simulink model "s06_sig_template_25"  (R2025b)
settings: Solver=ode4  StopTime=inf  FixedStep=P_sim_dt  EnableMultiTasking=on
InitFcn:
  | s06_data;
values from neighbouring files (symbols this model uses):
  P_c_locate_problist = ones(P_car_cnt, 1, 'single')    [s06_data.m]
  P_display_dt = 50e-3    (= 0.05)    [s06_data.m]
  P_dt = 25e-3    (= 0.025)    [s06_data.m]
  P_p_aMax = 1    [baseline_lqr_script.m]    (also in d71_data.m)
  P_p_Bf = 0.7    [d01_data.m]
  P_p_Br = 0.7    [d01_data.m]
  P_p_Cf = 2    [d01_data.m]
  P_p_Cr = 2    [d01_data.m]
  P_p_delta_max = 21.58/180*pi    (= 0.37664205258)    [d01_data.m]    (also in d71_data.m = 0.383972435439)
  P_p_deltan_max = 1    [d01_data.m]    (also in d71_data.m = 0.93)
  P_p_deltan_min = -P_p_deltan_max    (= -1)    [d01_data.m]    (also in d71_data.m = -0.93)
  P_p_Df = 2    [d01_data.m]
  P_p_Dr = 2.5    [d01_data.m]
  P_p_Ef = -0.1    [d01_data.m]
  P_p_EG = 0    [d01_data.m]    (also in d71_data.m = 0.02)
  P_p_Er = -0.05    [d01_data.m]
  P_p_J = 192e-6    (= 0.000192)    [d01_data.m]    (also in d71_data.m = 3e-06)
  P_p_k = 2.51    [d01_data.m]    (also in d71_data.m = 3.4)
  P_p_kd0 = 0.04    [d71_data.m]
  P_p_kd1 = 0.15    [d71_data.m]
  P_p_l = abs(P_p_frontaxle_1 + P_p_rearaxle_1)    [d01_data.m]    (also in d71_data.m = 0.0325)
  P_p_lf = P_p_frontaxle_1    (= 0.05)    [d01_data.m]    (also in d71_data.m = 0.01625)
  P_p_lr = P_p_rearaxle_1    (= 0.049)    [d01_data.m]    (also in d71_data.m = 0.01625)
  P_p_m = 132e-3    (= 0.132)    [d01_data.m]    (also in d71_data.m = 0.013)
  P_p_T = 316e-3    (= 0.316)    [d01_data.m]    (also in d71_data.m = 0.12)
  P_p_Tt = P_p_uTt + P_p_output_Tt    (= 0.11)    [d01_data.m]    (also in d71_data.m = 0.1)
  P_p_un_max = 1    [d01_data.m]    (also in d71_data.m = 0.2)
  P_p_un_min = -P_p_un_max    (= -1)    [d01_data.m]    (also in d71_data.m = -0.2)
  P_p_vRef = 0.2    [baseline_lqr_script.m]    (also in d71_data.m = 0.15)
  P_p_xvec0 = [ P_p_v0; P_p_s10; P_p_s20; P_p_psi0; 0; 0; 0 ]    [d01_data.m]    (also in d71_data.m)
  P_p_xvec1 = [ P_p_v0; P_p_s11; P_p_s21; P_p_psi1; 0; 0; 0 ]    [d01_data.m]    (also in d71_data.m)
  P_vfilter = single([ 0.0 0.0 ... (first row only)    [s06_data.m]
undefined symbols (not defined in the file or in its folder): CarInputsCmdForward, DiscIntNeverNeededParam, ManeuverTypePark, ManeuverTypePathFollow, mbc_car_display, P_cpseq, P_p, P_track
libraries: vrlib x2
(part 1 of 2)
settings Model: Creator=ftraenkle  LastModifiedBy=jossie
settings SolverCC: AlgebraicLoopSolver=TrustRegion
settings DataIOCC: LimitDataPoints=on  InspectSignalLogs=on  ReturnWorkspaceOutputs=off
settings OptimizationCC: DefaultParameterBehavior=Inlined  EnhancedBackFolding=on  PassReuseOutputArgsAs=Individual arguments  ExpressionDepthLimit=2147483647.0  ZeroExternalMemoryAtStartup=off  ZeroInternalMemoryAtStartup=off  OptimizeBlockOrder=speed  DifferentSizesBufferReuse=on  OptimizationCustomize=off  EfficientTunableParamExpr=on
settings DebuggingCC: SolverPrmCheckMsg=warning  ParameterTunabilityLossMsg=error  UnconnectedInputMsg=warning  UnconnectedOutputMsg=warning  UnconnectedLineMsg=warning  BusObjectLabelMismatch=error  AllowSymbolicDim=off  StateNameClashWarn=warning  SFUnexpectedBacktrackingDiag=warning  SFNoUnconditionalDefaultTransitionDiag=warning  SFExecutionAtInitializationDiag=none  ArithmeticOperatorsInVariantConditions=warning
settings HardwareCC: ProdBitPerLong=64.0  ProdHWDeviceType=Intel->x86-64 (Linux 64)
settings ModelReferenceCC: EnableRefExpFcnMdlSchedulingChecks=on
settings SFSimCC: SimUseLocalCustomCode=off  CustomCodeUndefinedFunction=UseInterfaceOnly
settings RTWCC: SystemTargetFile=ert.tlc  GenCodeOnly=on  PackageGeneratedCodeAndArtifacts=on  PackageName=d1.zip  TemplateMakefile=ert_default_tmf  GenerateReport=on  RTWUseLocalCustomCode=off  IncludeHyperlinkInReport=on  GenerateTraceInfo=on  GenerateTraceReportEml=on  GPUComputeCapability=3.5  DLArmComputeVersion=19.05  Description=Embedded Coder
settings CodeAppCC: ForceParamTrailComments=on  IgnoreCustomStorageClasses=off  OperatorAnnotations=on  SimulinkDataObjDesc=on  SFDataObjDesc=on  InsertBlockDesc=on
settings ERTTargetCC: RootIOFormat=Structure reference  DynamicArrayContainerType=coder::array  SupportVariableSizeSignals=on
settings ConfigComp: CovMetricSettings=dw  CovSaveCumulativeToWorkspaceVar=on  CovSaveSingleToWorkspaceVar=on  CovExternalEMLEnable=off

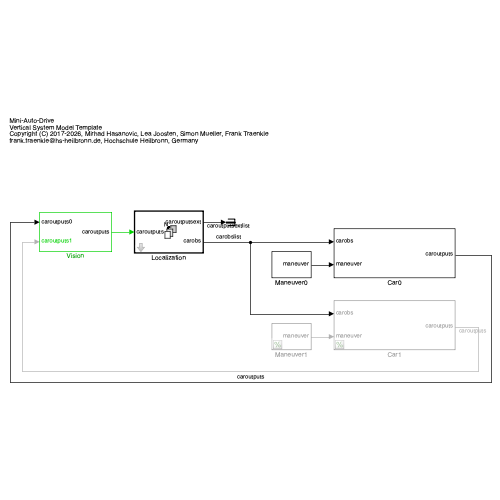
[thumbnail: Simulink's stored preview of the top-level diagram]
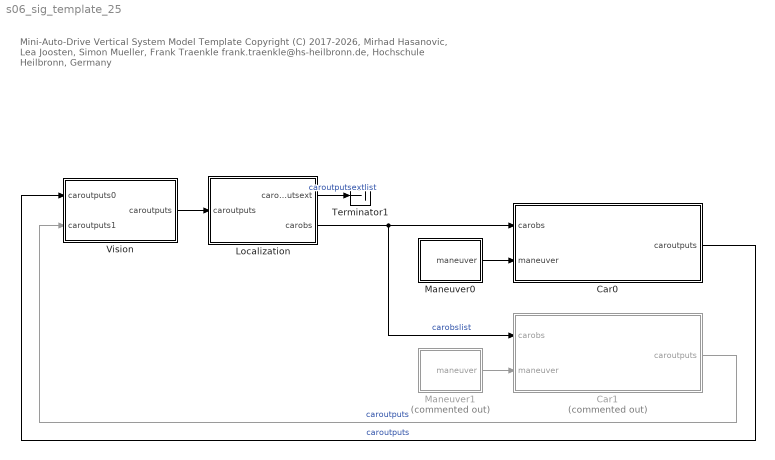
== system s06_sig_template_25 ==
  note: Mini-Auto-Drive
      | Vertical System Model Template
      | Copyright (C) 2017-2026, Mirhad Hasanovic, Lea Joosten, Simon Mueller, Frank Traenkle
      | frank.traenkle@hs-heilbronn.de, Hochschule Heilbronn, Germany
  Car0 : Subsystem
  Car1 : Subsystem  Commented=on
  Localization : Subsystem  TreatAsAtomicUnit=on  mask{P_mask_problist=P_c_locate_problist}
      mask prompts: P_mask_problist "Locate Probability"
  Maneuver0 : Subsystem
  Maneuver1 : Subsystem  Commented=on
  Terminator1 : Terminator
  Vision : Subsystem
  wires:
  Car0/1(caroutputs) -> Vision/1(caroutputs0)  "caroutputs"
  Localization/2(carobs) -> Car1/1(carobs), Car0/1(carobs)  "carobslist"
  Vision/1(caroutputs) -> Localization/1(caroutputs)
  Car1/1(caroutputs) -> Vision/2(caroutputs1)  "caroutputs"
  Maneuver0/1(maneuver) -> Car0/2(maneuver)
  Maneuver1/1(maneuver) -> Car1/2(maneuver)
  Localization/1(caroutputsext) -> Terminator1/1  "caroutputsextlist"

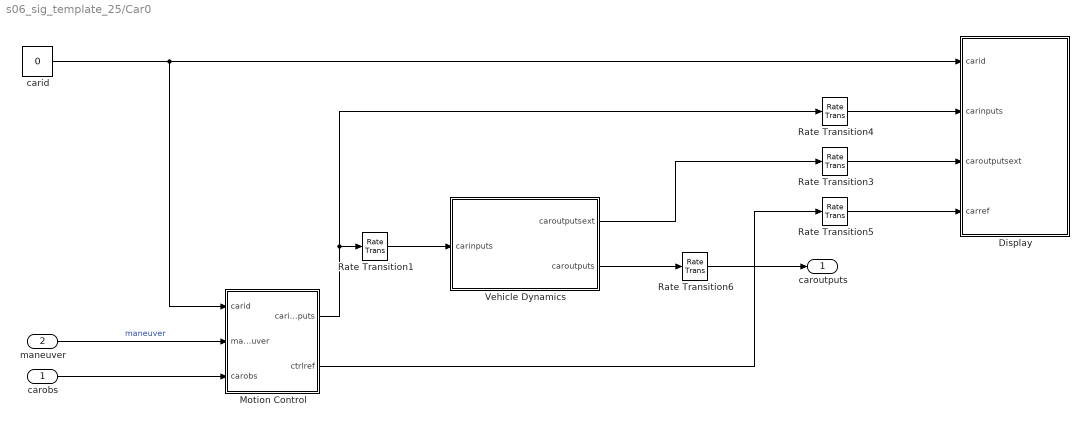
== system s06_sig_template_25/Car0 ==
  carobs : Inport  OutDataTypeStr=Bus: CAROBS
  maneuver : Inport  Port=2
  Display : Subsystem  TreatAsAtomicUnit=on  SystemSampleTime=P_display_dt
  Motion Control : Subsystem  TreatAsAtomicUnit=on
  Rate Transition1 : RateTransition  Integrity=off
  Rate Transition{3..6} (4 alike) : RateTransition
  Vehicle Dynamics : Subsystem  mask{P_mask_vec0=P_p_xvec0, P_mask_p=P_p(1)}
      mask prompts: P_mask_vec0 "Initial value"; P_mask_p "Parameters"
  carid : Constant  Value=0
  caroutputs : Outport  OutDataTypeStr=Bus: CAROUTPUTS
  wires:
  Vehicle Dynamics/1(caroutputsext) -> Rate Transition3/1
  Rate Transition5/1 -> Display/4(carref)
  Rate Transition3/1 -> Display/3(caroutputsext)
  Rate Transition4/1 -> Display/2(carinputs)
  Rate Transition1/1 -> Vehicle Dynamics/1(carinputs)
  Vehicle Dynamics/2(caroutputs) -> Rate Transition6/1
  Rate Transition6/1 -> caroutputs/1
  carid/1 -> Motion Control/1(carid), Display/1(carid)
  Motion Control/1(carinputs) -> Rate Transition4/1, Rate Transition1/1
  Motion Control/2(ctrlref) -> Rate Transition5/1
  carobs/1 -> Motion Control/3(carobs)
  maneuver/1 -> Motion Control/2(maneuver)  "maneuver"

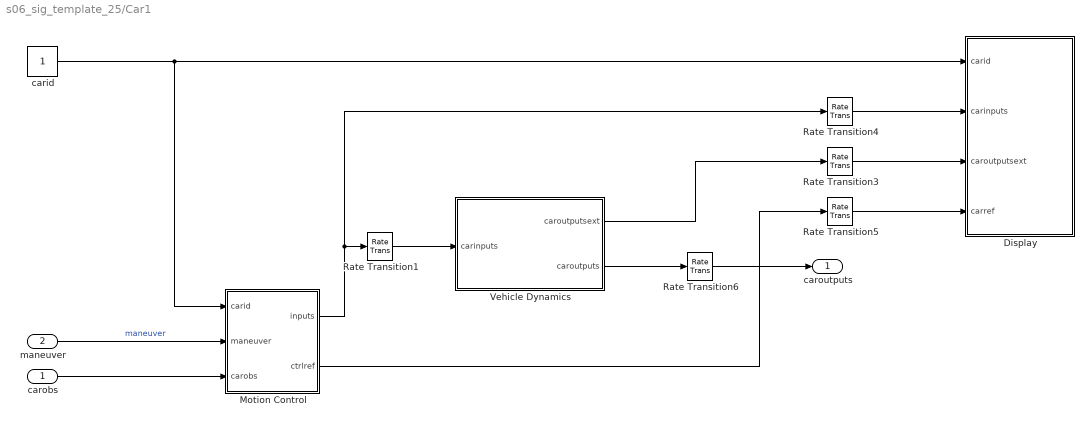
== system s06_sig_template_25/Car1 ==
  carobs : Inport  OutDataTypeStr=Bus: CAROBS
  maneuver : Inport  Port=2
  Display : Subsystem  TreatAsAtomicUnit=on  SystemSampleTime=P_display_dt
  Motion Control : Subsystem  TreatAsAtomicUnit=on  SystemSampleTime=P_dt
  Rate Transition{1,3..6} (5 alike) : RateTransition
  Vehicle Dynamics : Subsystem  mask{P_mask_vec0=P_p_xvec1, P_mask_p=P_p(1)}
      mask prompts: P_mask_vec0 "Initial value"; P_mask_p "Parameters"
  carid : Constant
  caroutputs : Outport  OutDataTypeStr=Bus: CAROUTPUTS
  wires:
  Vehicle Dynamics/1(caroutputsext) -> Rate Transition3/1
  Rate Transition5/1 -> Display/4(carref)
  Rate Transition3/1 -> Display/3(caroutputsext)
  Rate Transition4/1 -> Display/2(carinputs)
  Rate Transition1/1 -> Vehicle Dynamics/1(carinputs)
  Vehicle Dynamics/2(caroutputs) -> Rate Transition6/1
  Rate Transition6/1 -> caroutputs/1
  carid/1 -> Motion Control/1(carid), Display/1(carid)
  Motion Control/1(inputs) -> Rate Transition4/1, Rate Transition1/1
  Motion Control/2(ctrlref) -> Rate Transition5/1
  carobs/1 -> Motion Control/3(carobs)
  maneuver/1 -> Motion Control/2(maneuver)  "maneuver"

== system s06_sig_template_25/Localization ==
  caroutputs : Inport  Partition=on  PartitionDimension=1  PartitionWidth=1  PartitionOffset=0
  Constant : Constant  Value=true
  For Each : ForEach  DisableCoverage=on  IterateSubsysMaskParameter=on
  Locate : Subsystem
  caroutputsext : Outport  ConcatenationDimension=1
  carobs : Outport  Port=2  ConcatenationDimension=1
  wires:
  Locate/1(caroutputsext) -> caroutputsext/1
  Constant/1 -> Locate/Enable
  caroutputs/1 -> Locate/1(caroutputs)
  Locate/2(carobs) -> carobs/1

== system s06_sig_template_25/Maneuver0 ==
  Constant : Constant  Value=ManeuverTypePark
  Constant1 : Constant  Value=single(0.4)
  Constant2 : Constant  Value=single(2.0)
  Create Maneuver : MATLAB Function  TreatAsAtomicUnit=on
  maneuver : Outport
  wires:
  Constant/1 -> Create Maneuver/1(type)
  Constant1/1 -> Create Maneuver/2(vmax)
  Constant2/1 -> Create Maneuver/3(xref)
  Create Maneuver/1(maneuver) -> maneuver/1  "maneuver"

== system s06_sig_template_25/Maneuver1 ==
  Constant : Constant  Value=ManeuverTypePathFollow
  Constant1 : Constant  Value=single(0.5)
  Constant2 : Constant  Value=single(1.0)
  Create Maneuver : MATLAB Function  TreatAsAtomicUnit=on
  maneuver : Outport
  wires:
  Create Maneuver/1(maneuver) -> maneuver/1  "maneuver"
  Constant2/1 -> Create Maneuver/3(xref)
  Constant1/1 -> Create Maneuver/2(vmax)
  Constant/1 -> Create Maneuver/1(type)

== system s06_sig_template_25/Vision ==
  caroutputs0 : Inport  OutDataTypeStr=Bus:CAROUTPUTS
  caroutputs1 : Inport  Port=2  OutDataTypeStr=Bus:CAROUTPUTS
  Vector Concatenate : Concatenate  NumInputs=P_car_cnt
  caroutputs : Outport  OutDataTypeStr=Bus:CAROUTPUTS
  wires:
  Vector Concatenate/1 -> caroutputs/1  "caroutputs"
  caroutputs0/1 -> Vector Concatenate/1
  caroutputs1/1 -> Vector Concatenate/2

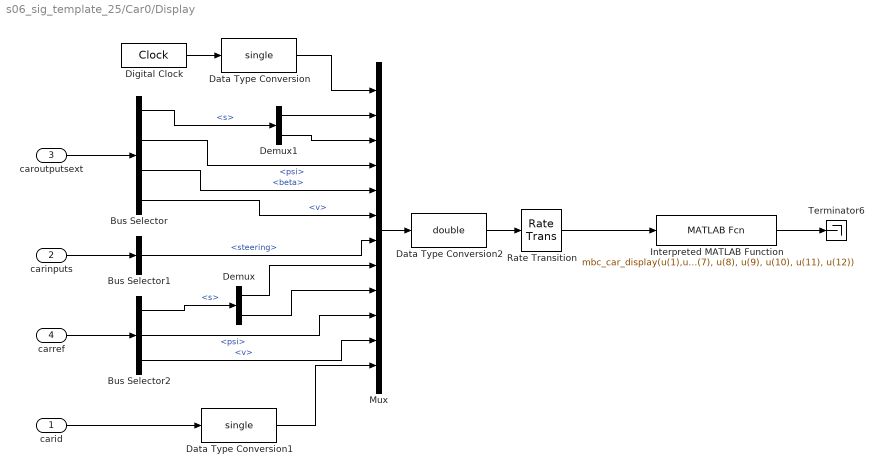
== system s06_sig_template_25/Car0/Display ==
  carid : Inport
  carinputs : Inport  Port=2
  caroutputsext : Inport  Port=3
  carref : Inport  Port=4
  Bus Selector : BusSelector  OutputSignals=s,psi,beta,v
  Bus Selector1 : BusSelector  OutputSignals=steering
  Bus Selector2 : BusSelector  OutputSignals=s,psi,v
  Data Type Conversion : DataTypeConversion  OutDataTypeStr=single  SaturateOnIntegerOverflow=off  RndMeth=Floor
  Data Type Conversion1 : DataTypeConversion  OutDataTypeStr=single  SaturateOnIntegerOverflow=off  RndMeth=Floor
  Data Type Conversion2 : DataTypeConversion  OutDataTypeStr=double  SaturateOnIntegerOverflow=off  RndMeth=Floor
  Demux : Demux  Outputs=2
  Demux1 : Demux  Outputs=2
  Digital Clock : DigitalClock  SampleTime=-1
  Interpreted MATLAB Function : MATLABFcn  MATLABFcn=mbc_car_display(u(1),u(2),u(3),u(4),u(5), u(6), u(7), u(8), u(9), u(10), u(11), u(12))
  Mux : Mux  Inputs=12
  Rate Transition : RateTransition  OutPortSampleTime=P_display_dt
  Terminator6 : Terminator
  wires:
  caroutputsext/1 -> Bus Selector/1
  Interpreted MATLAB Function/1 -> Terminator6/1
  Mux/1 -> Data Type Conversion2/1
  Rate Transition/1 -> Interpreted MATLAB Function/1
  Digital Clock/1 -> Data Type Conversion/1
  Bus Selector/2 -> Mux/4  "<psi>"
  carinputs/1 -> Bus Selector1/1
  Bus Selector1/1 -> Mux/7  "<steering>"
  Bus Selector/3 -> Mux/5  "<beta>"
  Bus Selector/4 -> Mux/6  "<v>"
  carref/1 -> Bus Selector2/1
  Bus Selector2/3 -> Mux/11  "<v>"
  Bus Selector2/2 -> Mux/10  "<psi>"
  Bus Selector2/1 -> Demux/1  "<s>"
  carid/1 -> Data Type Conversion1/1
  Data Type Conversion/1 -> Mux/1
  Data Type Conversion1/1 -> Mux/12
  Data Type Conversion2/1 -> Rate Transition/1
  Demux/1 -> Mux/8
  Demux/2 -> Mux/9
  Bus Selector/1 -> Demux1/1  "<s>"
  Demux1/1 -> Mux/2
  Demux1/2 -> Mux/3

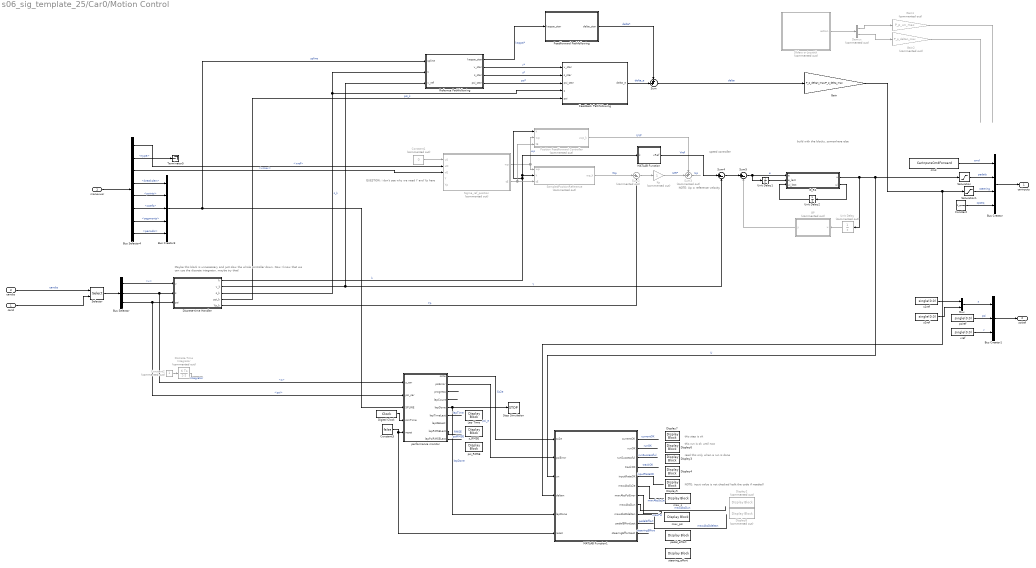
== system s06_sig_template_25/Car0/Motion Control ==
  note: Maybe this block is unnecessary and just slow the whole controller down. Now I know that we can use the discrete integrator, maybe try that!
  note: build with the blocks, somewhere else
  note: speed controller
  note: NOTE: Up = reference velocity
  note: QUESTION: i don't see why we need Y and Yp here
  note: read this only when a run is done
  note: NOTE: input value is not checked (edit the code if needed)
  note: this run is ok until now
  note: this step is ok
  carid : Inport
  maneuver : Inport  Port=2
  carobs : Inport  Port=3
  Bus Creator : BusCreator  Inputs=4  OutDataTypeStr=Bus: CARINPUTS  NonVirtualBus=on
  Bus Creator1 : BusCreator  Inputs=3  OutDataTypeStr=Bus: CTRLREFERENCE  NonVirtualBus=on
  Bus Creator3 : BusCreator  Inputs=5  OutDataTypeStr=Bus: SPLINE
  Bus Selector : BusSelector  OutputSignals=v,s,psi
  Bus Selector4 : BusSelector  OutputSignals=xref,type,vmax,breakslen,points,coefs,segments,periodic
  Constant : Constant  Value=P_cpseq  OutDataTypeStr=Bus: CHECKPOINTSEQUENCEMSG
  Constant1 : Constant  Commented=on  Value=0
  Constant2 : Constant  Commented=on
  Constant3 : Constant  Value=false
  Demux : Demux  Commented=on  Outputs=2
  Digital Clock : DigitalClock  SampleTime=P_dt
  Discrete-Time Integrator : DiscreteIntegrator  Commented=on  SampleTime=0.025  ICPrevOutput=DiscIntNeverNeededParam  ICPrevScaledInput=DiscIntNeverNeededParam
  Discrete-time Handler : MATLAB Function  TreatAsAtomicUnit=on
  Display2 : DisplayBlock  Commented=on  LabelPosition=Hide  Transparency=1  GridColor=[0.502, 0.502, 0.502]
  Display{3..7} (5 alike) : DisplayBlock  LabelPosition=Hide  Transparency=1  GridColor=[0.502, 0.502, 0.502]
  Display8 : DisplayBlock  Commented=on  LabelPosition=Hide  Transparency=1  GridColor=[0.502, 0.502, 0.502]
  Feedback Pathfollowing : MATLAB Function  TreatAsAtomicUnit=on
  Feedforward Pathfollowing : MATLAB Function  TreatAsAtomicUnit=on
  GP : MATLAB Function  Commented=on  TreatAsAtomicUnit=on
  G_R1 : MATLAB Function  TreatAsAtomicUnit=on
  Gain : Gain  Gain=P_p_deltan_max/P_p_delta_max
  Gain1 : Gain  Commented=on  Gain=P_p_un_max
  Gain2 : Gain  Commented=on  Gain=P_p_deltan_max
  Kp : Gain  Commented=on
  Lap Time : DisplayBlock  LabelPosition=Hide  Transparency=1  GridColor=[0.502, 0.502, 0.502]
  MATLAB Function : MATLAB Function  TreatAsAtomicUnit=on
  MATLAB Function1 : MATLAB Function  TreatAsAtomicUnit=on
  Mux : Mux  Inputs=2
  Position Feedforward Controller : MATLAB Function  Commented=on  TreatAsAtomicUnit=on
  Refernce Pathfollowing : MATLAB Function  TreatAsAtomicUnit=on
  SampledPositionReference : MATLAB Function  Commented=on  TreatAsAtomicUnit=on
  Saturation : Saturate  UpperLimit=P_p_un_max  LowerLimit=P_p_un_min
  Saturation1 : Saturate  UpperLimit=P_p_deltan_max  LowerLimit=P_p_deltan_min
  Selector : Selector  IndexMode=Zero-based  InputPortWidth=P_car_cnt  IndexOptions=Index vector (port)  Indices=0  OutputSizes=1
  Sigma_ref_position : MATLAB Function  Commented=on  TreatAsAtomicUnit=on
  Sliders or Joystick : Subsystem  Commented=on  Variant=on  VariantControlMode=label  LabelModeActiveChoice=true
  Stop Simulation : Stop
  Sum : Sum  Inputs=++|
  Sum2 : Sum  Commented=on  Inputs=|+-
  Sum3 : Sum  Commented=on  Inputs=++|
  Sum4 : Sum  Inputs=|+-
  Sum5 : Sum  Inputs=|+-
  Terminator5 : Terminator
  Unit Delay : UnitDelay  Commented=on  SampleTime=-1
  Unit Delay1 : UnitDelay  SampleTime=-1
  Unit Delay2 : UnitDelay  SampleTime=-1
  cmd : Constant  Value=CarInputsCmdForward
  max_psi : DisplayBlock  LabelPosition=Hide  Transparency=1  GridColor=[0.502, 0.502, 0.502]
  max_s : DisplayBlock  LabelPosition=Hide  Transparency=1  GridColor=[0.502, 0.502, 0.502]
  pedal_effort : DisplayBlock  LabelPosition=Hide  Transparency=1  GridColor=[0.502, 0.502, 0.502]
  performance monitor : MATLAB Function  TreatAsAtomicUnit=on
  psi_RMSE : DisplayBlock  LabelPosition=Hide  Transparency=1  GridColor=[0.502, 0.502, 0.502]
  psiref : Constant  Value=single(0.0)
  s1ref : Constant  Value=single(0.0)
  s2ref : Constant  Value=single(0.0)
  s_RMSE : DisplayBlock  LabelPosition=Hide  Transparency=1  GridColor=[0.502, 0.502, 0.502]
  steering_effort : DisplayBlock  LabelPosition=Hide  Transparency=1  GridColor=[0.502, 0.502, 0.502]
  vref : Constant  Value=single(0.0)
  carinputs : Outport  VectorParamsAs1DForOutWhenUnconnected=off
  ctrlref : Outport  Port=2  VectorParamsAs1DForOutWhenUnconnected=off
  wires:
  Bus Creator1/1 -> ctrlref/1
  vref/1 -> Bus Creator1/3  "v"
  Bus Selector/2 -> performance monitor/1(s_car), Discrete-time Handler/2(s)  "<s>"
  Mux/1 -> Bus Creator1/1  "s"
  Bus Selector4/7 -> Bus Creator3/4  "<segments>"
  Bus Selector4/5 -> Bus Creator3/2  "<points>"
  Bus Selector4/6 -> Bus Creator3/3  "<coefs>"
  Bus Selector4/8 -> Bus Creator3/5  "<periodic>"
  Bus Selector4/2 -> Terminator5/1  "<type>"
  Bus Selector4/4 -> Bus Creator3/1  "<breakslen>"
  maneuver/1 -> Bus Selector4/1
  carid/1 -> Selector/2
  carobs/1 -> Selector/1  "carobs"
  Selector/1 -> Bus Selector/1
  Bus Selector4/1 -> Sigma_ref_position/2(xD)  "<xref>"
  Bus Selector4/3 -> Sigma_ref_position/3(vE)  "<vmax>"
  Bus Selector/1 -> Discrete-time Handler/1(v)  "<v>"
  Bus Selector/3 -> performance monitor/2(psi_car), Discrete-time Handler/3(psi)  "<psi>"
  s1ref/1 -> Mux/1
  s2ref/1 -> Mux/2
  psiref/1 -> Bus Creator1/2  "psi"
  Demux/1 -> Gain1/1
  Constant/1 -> Bus Creator/4  "cpseq"
  Bus Creator/1 -> carinputs/1
  cmd/1 -> Bus Creator/1  "cmd"
  Gain1/1 -> ?
  Saturation1/1 -> Bus Creator/3  "steering"
  Sliders or Joystick/1(action) -> Demux/1
  Demux/2 -> Gain2/1
  Gain2/1 -> ?
  Saturation/1 -> Bus Creator/2  "pedals"
  Bus Creator3/1 -> performance monitor/3(SPLINE), Refernce Pathfollowing/1(spline)  "spline"
  Constant1/1 -> Sigma_ref_position/1(v0)
  SampledPositionReference/1(wp_k) -> Sum2/1  "Wp"
  Sigma_ref_position/1(wp) -> Position Feedforward Controller/2(wp), SampledPositionReference/1(wp)  "wp"
  Discrete-time Handler/1(k) -> MATLAB Function/1(k), SampledPositionReference/2(k), Position Feedforward Controller/1(k)  "k"
  Discrete-time Handler/5(Yp_k) -> Sum2/2  "Yp"
  Sum2/1 -> Kp/1
  Kp/1 -> Sum3/2  "URP"
  Sum3/1 -> ?  "Up"
  Position Feedforward Controller/1(uvp_k) -> Sum3/1  "UVP"
  Discrete-time Handler/2(v_k) -> Refernce Pathfollowing/3(v_ref), Sum4/2  "Y"
  Sum4/1 -> Sum5/1
  GP/1(y) -> Sum5/2
  Sum5/1 -> Unit Delay1/1, G_R1/1(e)  "e"
  Unit Delay1/1 -> G_R1/2(e_last)
  G_R1/2(ui) -> Unit Delay2/1
  Unit Delay2/1 -> G_R1/3(ui_last)
  Feedforward Pathfollowing/1(delta_star) -> Sum/1  "delta*"
  Feedback Pathfollowing/1(delta_e) -> Sum/2  "delta_e"
  Refernce Pathfollowing/1(kappa_star) -> Feedforward Pathfollowing/1(kappa_star)  "kappa*"
  Refernce Pathfollowing/2(v_star) -> Feedback Pathfollowing/1(v_star)  "v*"
  Refernce Pathfollowing/3(s_star) -> Feedback Pathfollowing/2(s_star)  "s*"
  Refernce Pathfollowing/4(psi_star) -> Feedback Pathfollowing/3(psi_star)  "psi*"
  Discrete-time Handler/3(s_k) -> Refernce Pathfollowing/2(s), Feedback Pathfollowing/4(s)  "s_k"
  Discrete-time Handler/4(psi_k) -> Feedback Pathfollowing/5(psi)  "psi_k"
  Sum/1 -> Gain/1  "delta"
  Unit Delay/1 -> GP/1(u)
  Constant2/1 -> Discrete-Time Integrator/1
  Discrete-Time Integrator/1 -> ?  "integrator"
  Sigma_ref_position/2(tE) -> SampledPositionReference/3(tE), Position Feedforward Controller/3(tE)
  Gain/1 -> MATLAB Function1/4(deltan), Saturation1/1
  MATLAB Function/1(vRef) -> Sum4/1  "Vref"
  MATLAB Function1/9(maxAbsDdeltan) -> ?  "maxAbsDdeltan"
  MATLAB Function1/8(maxAbsDun) -> ?  "maxAbsDun"
  Constant3/1 -> MATLAB Function1/6(reset), performance monitor/5(reset)
  performance monitor/5(lapDone) -> Stop Simulation/1, MATLAB Function1/5(lapDone)  "lapDone"
  G_R1/1(u) -> Saturation/1, MATLAB Function1/3(un), Unit Delay/1  "U"
  MATLAB Function1/3(runSuccessful) -> ?  "runSuccessful"
  performance monitor/1(sc2e) -> MATLAB Function1/1(sc2e)  "Sc2e"
  performance monitor/2(psiError) -> MATLAB Function1/2(psiError)  "psi_e"
  performance monitor/9(lapPsiRMSELast) -> ?  "psiRMSE"
  MATLAB Function1/2(runOK) -> ?  "runOK"
  MATLAB Function1/10(pedalEffortLast) -> ?  "pedalEffort"
  MATLAB Function1/11(steeringEffortLast) -> ?  "steeringEffort"
  MATLAB Function1/7(maxAbsPsiError) -> ?  "maxPsi"
  MATLAB Function1/1(currentOK) -> ?  "currentOK"
  Digital Clock/1 -> performance monitor/4(simTime)
  MATLAB Function1/5(inputRateOK) -> ?  "inputRateOK"
  performance monitor/4(lapCount) -> ?
  MATLAB Function1/4(trackOK) -> ?  "trackOK"
  MATLAB Function1/6(maxAbsSc2e) -> ?  "maxAbsSc2e"
  performance monitor/6(lapTimeLast) -> ?  "lapTime"
  performance monitor/3(progress) -> ?
  performance monitor/8(lapRMSELast) -> ?  "RMSE"

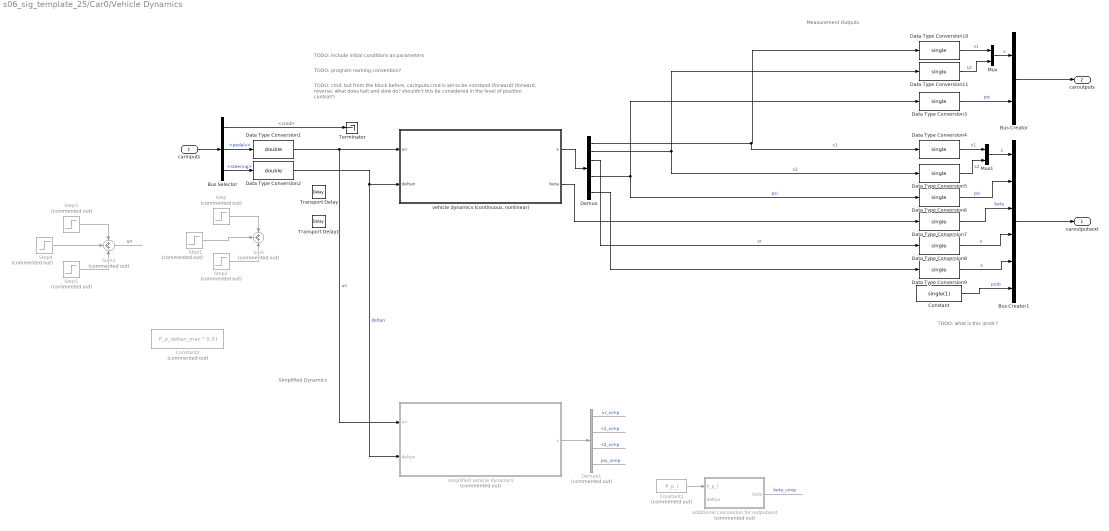
== system s06_sig_template_25/Car0/Vehicle Dynamics ==
  note: Simplified Dynamics
  note: TODO: cmd, but from the block before, carinputs.cmd is set to be constand (forward)
      | (forward, reverse, what does halt and slow do? shouldn't this be considered in the level of position control?)
  note: TODO: what is this 'prob'?
  note: TODO: program naming convention?
  note: TODO: include initial conditions as parameters
  note: Measurement Outputs
  carinputs : Inport
  Bus Creator : BusCreator  Inputs=2  OutDataTypeStr=Bus: CAROUTPUTS  NonVirtualBus=on
  Bus Creator1 : BusCreator  Inputs=6  OutDataTypeStr=Bus: CAROUTPUTSEXT  NonVirtualBus=on
  Bus Selector : BusSelector  OutputSignals=cmd,pedals,steering
  Constant : Constant  Value=single(1)
  Constant1 : Constant  Commented=on  Value=P_p_l
  Constant2 : Constant  Commented=on  Value=P_p_deltan_max * 0.01
  Data Type Conversion1 : DataTypeConversion  OutDataTypeStr=double  SaturateOnIntegerOverflow=off  RndMeth=Floor
  Data Type Conversion{3..11} (9 alike) : DataTypeConversion  OutDataTypeStr=single  SaturateOnIntegerOverflow=off  RndMeth=Floor
  Data Type Conversion2 : DataTypeConversion  OutDataTypeStr=double  SaturateOnIntegerOverflow=off  RndMeth=Floor
  Demux : Demux  Outputs=7
  Demux1 : Demux  Commented=on
  Mux : Mux  Inputs=2
  Mux1 : Mux  Inputs=2
  Step : Step  Commented=on  Time=0  After=P_p_un_max*0.5  SampleTime=0
  Step1 : Step  Commented=on  After=-P_p_un_max*0.5  SampleTime=0
  Step2 : Step  Commented=on  Time=2  After=P_p_un_max  SampleTime=0
  Step3 : Step  Commented=on  Time=0  After=P_p_un_max  SampleTime=0
  Step4 : Step  Commented=on  After=-2*P_p_un_max  SampleTime=0
  Step5 : Step  Commented=on  Time=2  After=P_p_un_max  SampleTime=0
  Sum : Sum  Commented=on  Inputs=+++
  Sum1 : Sum  Commented=on  Inputs=+++
  Terminator : Terminator
  Transport Delay : TransportDelay  DelayTime=P_p_Tt
  Transport Delay1 : TransportDelay  DelayTime=P_p_Tt
  additional calculation for outputsext : MATLAB Function  Commented=on  TreatAsAtomicUnit=on
  simplified vehicle dynamics : Subsystem  Commented=on
  "vehicle dynamics (continuous, nonlinear)" : Subsystem
  caroutputsext : Outport  OutDataTypeStr=Bus: CAROUTPUTSEXT  VectorParamsAs1DForOutWhenUnconnected=off
  caroutputs : Outport  Port=2  OutDataTypeStr=Bus: CAROUTPUTS  VectorParamsAs1DForOutWhenUnconnected=off
  wires:
  Bus Selector/2 -> Data Type Conversion1/1  "<pedals>"
  Bus Selector/3 -> Data Type Conversion2/1  "<steering>"
  Bus Creator/1 -> caroutputs/1
  Bus Creator1/1 -> caroutputsext/1
  Bus Selector/1 -> Terminator/1  "<cmd>"
  Mux1/1 -> Bus Creator1/1  "s"
  Data Type Conversion5/1 -> Mux1/2  "s2"
  Data Type Conversion4/1 -> Mux1/1  "s1"
  Mux/1 -> Bus Creator/1  "s"
  Data Type Conversion9/1 -> Bus Creator1/5  "x"
  Data Type Conversion8/1 -> Bus Creator1/4  "v"
  Data Type Conversion7/1 -> Bus Creator1/3  "beta"
  Data Type Conversion6/1 -> Bus Creator1/2  "psi"
  Data Type Conversion3/1 -> Bus Creator/2  "psi"
  Data Type Conversion11/1 -> Mux/2  "s2"
  Data Type Conversion10/1 -> Mux/1  "s1"
  Constant/1 -> Bus Creator1/6  "prob"
  "vehicle dynamics (continuous, nonlinear)"/1(x) -> Demux/1
  Demux/1 -> Data Type Conversion4/1, Data Type Conversion10/1  "s1"
  Demux/2 -> Data Type Conversion5/1, Data Type Conversion11/1  "s2"
  Demux/5 -> Data Type Conversion6/1, Data Type Conversion3/1  "psi"
  "vehicle dynamics (continuous, nonlinear)"/2(beta) -> Data Type Conversion7/1
  Demux/7 -> Data Type Conversion9/1
  Demux/3 -> Data Type Conversion8/1  "vr"
  simplified vehicle dynamics/1(x) -> Demux1/1
  Demux1/1 -> ?  "vr_simp"
  Constant1/1 -> additional calculation for outputsext/1(P_p_l)
  Demux1/2 -> ?  "s1_simp"
  Demux1/3 -> ?  "s2_simp"
  Demux1/4 -> ?  "psi_simp"
  additional calculation for outputsext/1(beta) -> ?  "beta_simp"
  Step/1 -> Sum/1
  Step1/1 -> Sum/2
  Data Type Conversion1/1 -> simplified vehicle dynamics/1(un), "vehicle dynamics (continuous, nonlinear)"/1(un)  "un"
  Data Type Conversion2/1 -> simplified vehicle dynamics/2(deltan), "vehicle dynamics (continuous, nonlinear)"/2(deltan)  "deltan"
  Step2/1 -> Sum/3
  Step4/1 -> Sum1/2
  Step5/1 -> Sum1/3
  Step3/1 -> Sum1/1
  Sum1/1 -> ?  "un"
  carinputs/1 -> Bus Selector/1

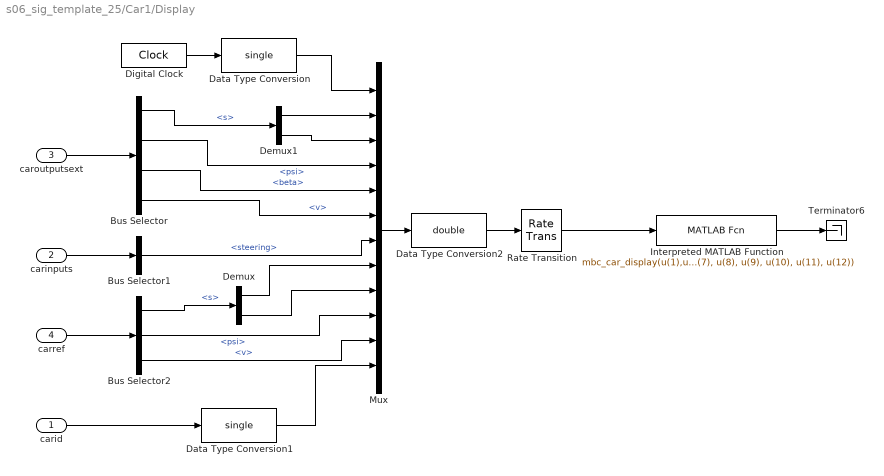
== system s06_sig_template_25/Car1/Display ==
  carid : Inport
  carinputs : Inport  Port=2
  caroutputsext : Inport  Port=3
  carref : Inport  Port=4
  Bus Selector : BusSelector  OutputSignals=s,psi,beta,v
  Bus Selector1 : BusSelector  OutputSignals=steering
  Bus Selector2 : BusSelector  OutputSignals=s,psi,v
  Data Type Conversion : DataTypeConversion  OutDataTypeStr=single  SaturateOnIntegerOverflow=off  RndMeth=Floor
  Data Type Conversion1 : DataTypeConversion  OutDataTypeStr=single  SaturateOnIntegerOverflow=off  RndMeth=Floor
  Data Type Conversion2 : DataTypeConversion  OutDataTypeStr=double  SaturateOnIntegerOverflow=off  RndMeth=Floor
  Demux : Demux  Outputs=2
  Demux1 : Demux  Outputs=2
  Digital Clock : DigitalClock  SampleTime=-1
  Interpreted MATLAB Function : MATLABFcn  MATLABFcn=mbc_car_display(u(1),u(2),u(3),u(4),u(5), u(6), u(7), u(8), u(9), u(10), u(11), u(12))
  Mux : Mux  Inputs=12
  Rate Transition : RateTransition  OutPortSampleTime=P_display_dt
  Terminator6 : Terminator
  wires:
  caroutputsext/1 -> Bus Selector/1
  Interpreted MATLAB Function/1 -> Terminator6/1
  Mux/1 -> Data Type Conversion2/1
  Rate Transition/1 -> Interpreted MATLAB Function/1
  Digital Clock/1 -> Data Type Conversion/1
  Bus Selector/2 -> Mux/4  "<psi>"
  carinputs/1 -> Bus Selector1/1
  Bus Selector1/1 -> Mux/7  "<steering>"
  Bus Selector/3 -> Mux/5  "<beta>"
  Bus Selector/4 -> Mux/6  "<v>"
  carref/1 -> Bus Selector2/1
  Bus Selector2/3 -> Mux/11  "<v>"
  Bus Selector2/2 -> Mux/10  "<psi>"
  Bus Selector2/1 -> Demux/1  "<s>"
  carid/1 -> Data Type Conversion1/1
  Data Type Conversion/1 -> Mux/1
  Data Type Conversion1/1 -> Mux/12
  Data Type Conversion2/1 -> Rate Transition/1
  Demux/1 -> Mux/8
  Demux/2 -> Mux/9
  Bus Selector/1 -> Demux1/1  "<s>"
  Demux1/1 -> Mux/2
  Demux1/2 -> Mux/3

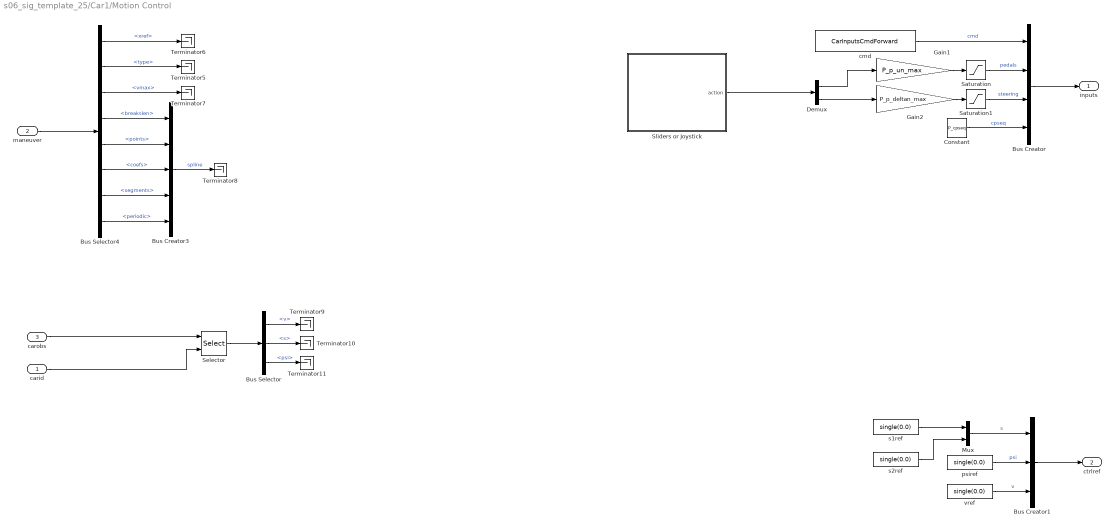
== system s06_sig_template_25/Car1/Motion Control ==
  carid : Inport
  maneuver : Inport  Port=2
  carobs : Inport  Port=3
  Bus Creator : BusCreator  Inputs=4  OutDataTypeStr=Bus: CARINPUTS  NonVirtualBus=on
  Bus Creator1 : BusCreator  Inputs=3  OutDataTypeStr=Bus: CTRLREFERENCE  NonVirtualBus=on
  Bus Creator3 : BusCreator  Inputs=5  OutDataTypeStr=Bus: SPLINE
  Bus Selector : BusSelector  OutputSignals=v,s,psi
  Bus Selector4 : BusSelector  OutputSignals=xref,type,vmax,breakslen,points,coefs,segments,periodic
  Constant : Constant  Value=P_cpseq  OutDataTypeStr=Bus: CHECKPOINTSEQUENCEMSG
  Demux : Demux  Outputs=2
  Gain1 : Gain  Gain=P_p_un_max
  Gain2 : Gain  Gain=P_p_deltan_max
  Mux : Mux  Inputs=2
  Saturation : Saturate  UpperLimit=P_p_un_max  LowerLimit=P_p_un_min
  Saturation1 : Saturate  UpperLimit=P_p_deltan_max  LowerLimit=P_p_deltan_min
  Selector : Selector  IndexMode=Zero-based  InputPortWidth=P_car_cnt  IndexOptions=Index vector (port)  Indices=0  OutputSizes=1
  Sliders or Joystick : Subsystem  Variant=on  VariantControlMode=label  LabelModeActiveChoice=true
  Terminator{5..11} (7 alike) : Terminator
  cmd : Constant  Value=CarInputsCmdForward
  psiref : Constant  Value=single(0.0)
  s1ref : Constant  Value=single(0.0)
  s2ref : Constant  Value=single(0.0)
  vref : Constant  Value=single(0.0)
  inputs : Outport  VectorParamsAs1DForOutWhenUnconnected=off
  ctrlref : Outport  Port=2  VectorParamsAs1DForOutWhenUnconnected=off
  wires:
  Bus Creator1/1 -> ctrlref/1
  vref/1 -> Bus Creator1/3  "v"
  Bus Selector/2 -> Terminator10/1  "<s>"
  Mux/1 -> Bus Creator1/1  "s"
  Bus Selector4/7 -> Bus Creator3/4  "<segments>"
  Bus Selector4/5 -> Bus Creator3/2  "<points>"
  Bus Selector4/6 -> Bus Creator3/3  "<coefs>"
  Bus Selector4/8 -> Bus Creator3/5  "<periodic>"
  Bus Selector4/2 -> Terminator5/1  "<type>"
  Bus Selector4/4 -> Bus Creator3/1  "<breakslen>"
  maneuver/1 -> Bus Selector4/1
  carid/1 -> Selector/2
  carobs/1 -> Selector/1
  Selector/1 -> Bus Selector/1
  Bus Selector4/1 -> Terminator6/1  "<xref>"
  Bus Selector4/3 -> Terminator7/1  "<vmax>"
  Bus Creator3/1 -> Terminator8/1  "spline"
  Bus Selector/1 -> Terminator9/1  "<v>"
  Bus Selector/3 -> Terminator11/1  "<psi>"
  s1ref/1 -> Mux/1
  s2ref/1 -> Mux/2
  psiref/1 -> Bus Creator1/2  "psi"
  Saturation/1 -> Bus Creator/2  "pedals"
  Demux/1 -> Gain1/1
  Constant/1 -> Bus Creator/4  "cpseq"
  Bus Creator/1 -> inputs/1
  cmd/1 -> Bus Creator/1  "cmd"
  Gain1/1 -> Saturation/1
  Saturation1/1 -> Bus Creator/3  "steering"
  Sliders or Joystick/1(action) -> Demux/1
  Demux/2 -> Gain2/1
  Gain2/1 -> Saturation1/1

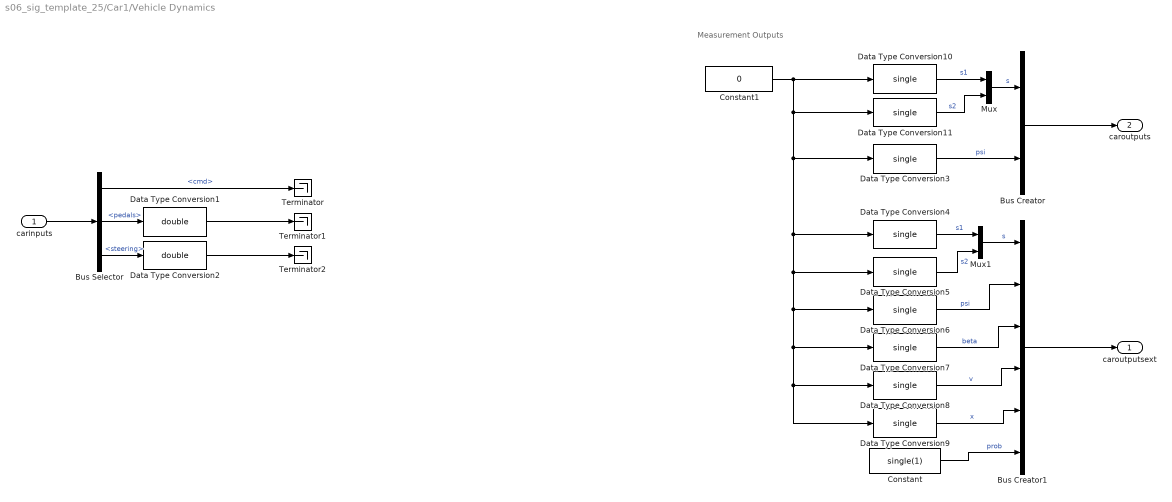
== system s06_sig_template_25/Car1/Vehicle Dynamics ==
  note: Measurement Outputs
  carinputs : Inport
  Bus Creator : BusCreator  Inputs=2  OutDataTypeStr=Bus: CAROUTPUTS  NonVirtualBus=on
  Bus Creator1 : BusCreator  Inputs=6  OutDataTypeStr=Bus: CAROUTPUTSEXT  NonVirtualBus=on
  Bus Selector : BusSelector  OutputSignals=cmd,pedals,steering
  Constant : Constant  Value=single(1)
  Constant1 : Constant  Value=0
  Data Type Conversion1 : DataTypeConversion  OutDataTypeStr=double  SaturateOnIntegerOverflow=off  RndMeth=Floor
  Data Type Conversion{3..11} (9 alike) : DataTypeConversion  OutDataTypeStr=single  SaturateOnIntegerOverflow=off  RndMeth=Floor
  Data Type Conversion2 : DataTypeConversion  OutDataTypeStr=double  SaturateOnIntegerOverflow=off  RndMeth=Floor
  Mux : Mux  Inputs=2
  Mux1 : Mux  Inputs=2
  Terminator : Terminator
  Terminator1 : Terminator
  Terminator2 : Terminator
  caroutputsext : Outport  OutDataTypeStr=Bus: CAROUTPUTSEXT  VectorParamsAs1DForOutWhenUnconnected=off
  caroutputs : Outport  Port=2  OutDataTypeStr=Bus: CAROUTPUTS  VectorParamsAs1DForOutWhenUnconnected=off
  wires:
  carinputs/1 -> Bus Selector/1
  Bus Selector/2 -> Data Type Conversion1/1  "<pedals>"
  Bus Selector/3 -> Data Type Conversion2/1  "<steering>"
  Bus Creator/1 -> caroutputs/1
  Bus Creator1/1 -> caroutputsext/1
  Bus Selector/1 -> Terminator/1  "<cmd>"
  Data Type Conversion1/1 -> Terminator1/1
  Data Type Conversion2/1 -> Terminator2/1
  Constant1/1 -> Data Type Conversion9/1, Data Type Conversion8/1, Data Type Conversion7/1, Data Type Conversion6/1, Data Type Conversion5/1, Data Type Conversion4/1, Data Type Conversion3/1, Data Type Conversion11/1, Data Type Conversion10/1
  Mux1/1 -> Bus Creator1/1  "s"
  Data Type Conversion5/1 -> Mux1/2  "s2"
  Data Type Conversion4/1 -> Mux1/1  "s1"
  Mux/1 -> Bus Creator/1  "s"
  Data Type Conversion9/1 -> Bus Creator1/5  "x"
  Data Type Conversion8/1 -> Bus Creator1/4  "v"
  Data Type Conversion7/1 -> Bus Creator1/3  "beta"
  Data Type Conversion6/1 -> Bus Creator1/2  "psi"
  Data Type Conversion3/1 -> Bus Creator/2  "psi"
  Data Type Conversion11/1 -> Mux/2  "s2"
  Data Type Conversion10/1 -> Mux/1  "s1"
  Constant/1 -> Bus Creator1/6  "prob"

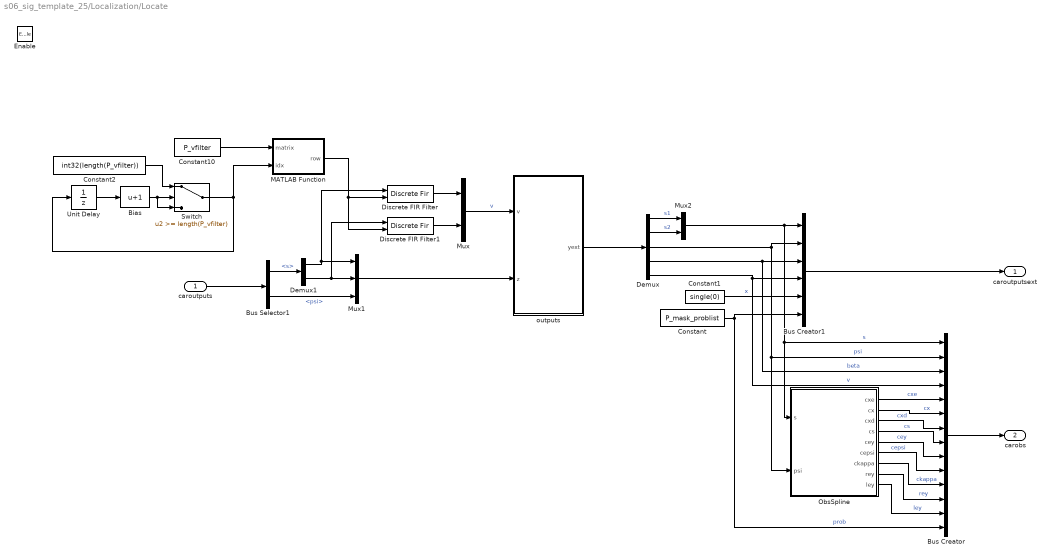
== system s06_sig_template_25/Localization/Locate ==
  caroutputs : Inport
  Enable : EnablePort
  Bias : Bias  Bias=1  SaturateOnIntegerOverflow=off
  Bus Creator : BusCreator  Inputs=14  OutDataTypeStr=Bus: CAROBS  NonVirtualBus=on
  Bus Creator1 : BusCreator  Inputs=6  OutDataTypeStr=Bus: CAROUTPUTSEXT  NonVirtualBus=on
  Bus Selector1 : BusSelector  OutputSignals=s,psi
  Constant : Constant  Value=P_mask_problist
  Constant1 : Constant  Value=single(0)
  Constant10 : Constant  Value=P_vfilter
  Constant2 : Constant  Value=int32(length(P_vfilter))
  Demux : Demux  Outputs=5
  Demux1 : Demux  Outputs=2
  Discrete FIR Filter : DiscreteFir  CoefSource=Input port
      settings: InputPortMap=u0,u1
  Discrete FIR Filter1 : DiscreteFir  CoefSource=Input port
      settings: InputPortMap=u0,u1
  MATLAB Function : MATLAB Function  TreatAsAtomicUnit=on
  Mux : Mux  Inputs=2
  Mux1 : Mux  Inputs=3
  Mux2 : Mux  Inputs=2
  ObsSpline : Subsystem
  Switch : Switch  Threshold=length(P_vfilter)  SaturateOnIntegerOverflow=off  InputSameDT=off
  Unit Delay : UnitDelay  InitialCondition=int32(0)  SampleTime=-1
  outputs : MATLAB Function  TreatAsAtomicUnit=on  SystemSampleTime=P_dt
  caroutputsext : Outport
  carobs : Outport  Port=2
  wires:
  Mux1/1 -> outputs/2(z)
  Bus Selector1/2 -> Mux1/3  "<psi>"
  MATLAB Function/1(row) -> Discrete FIR Filter1/2, Discrete FIR Filter/2
  Discrete FIR Filter1/1 -> Mux/2
  Discrete FIR Filter/1 -> Mux/1
  Constant/1 -> Bus Creator/14, Bus Creator1/6  "prob"
  Bus Selector1/1 -> Demux1/1  "<s>"
  Demux1/2 -> Discrete FIR Filter1/1, Mux1/2
  Demux/4 -> Bus Creator/3, Bus Creator1/3  "beta"
  Mux2/1 -> ObsSpline/1(s), Bus Creator/1, Bus Creator1/1  "s"
  caroutputs/1 -> Bus Selector1/1
  Constant1/1 -> Bus Creator1/5  "x"
  Demux/1 -> Mux2/1  "s1"
  Demux/2 -> Mux2/2  "s2"
  Demux1/1 -> Discrete FIR Filter/1, Mux1/1
  Bus Creator1/1 -> caroutputsext/1
  Demux/5 -> Bus Creator/4, Bus Creator1/4  "v"
  Mux/1 -> outputs/1(v)  "v"
  outputs/1(yext) -> Demux/1
  Demux/3 -> ObsSpline/2(psi), Bus Creator/2, Bus Creator1/2  "psi"
  Constant10/1 -> MATLAB Function/1(matrix)
  Switch/1 -> Unit Delay/1, MATLAB Function/2(idx)
  Unit Delay/1 -> Bias/1
  Bias/1 -> Switch/3, Switch/2
  Constant2/1 -> Switch/1
  ObsSpline/1(cxe) -> Bus Creator/5  "cxe"
  ObsSpline/2(cx) -> Bus Creator/6  "cx"
  ObsSpline/3(cxd) -> Bus Creator/7  "cxd"
  ObsSpline/5(cey) -> Bus Creator/9  "cey"
  ObsSpline/6(cepsi) -> Bus Creator/10  "cepsi"
  ObsSpline/7(ckappa) -> Bus Creator/11  "ckappa"
  ObsSpline/8(rey) -> Bus Creator/12  "rey"
  ObsSpline/9(ley) -> Bus Creator/13  "ley"
  Bus Creator/1 -> carobs/1
  ObsSpline/4(cs) -> Bus Creator/8  "cs"

== system s06_sig_template_25/Car0/Motion Control/Sliders or Joystick ==
  note: 1) Add Subsystem or Model blocks as valid variant choices.
      | 2) You cannot connect blocks at this level. At simulation, connectivity is automatically
      | determined, based on the active variant and port name matching.
  Joystick : Subsystem  VariantControl=false
  Sliders : Subsystem  VariantControl=true
  action : Outport

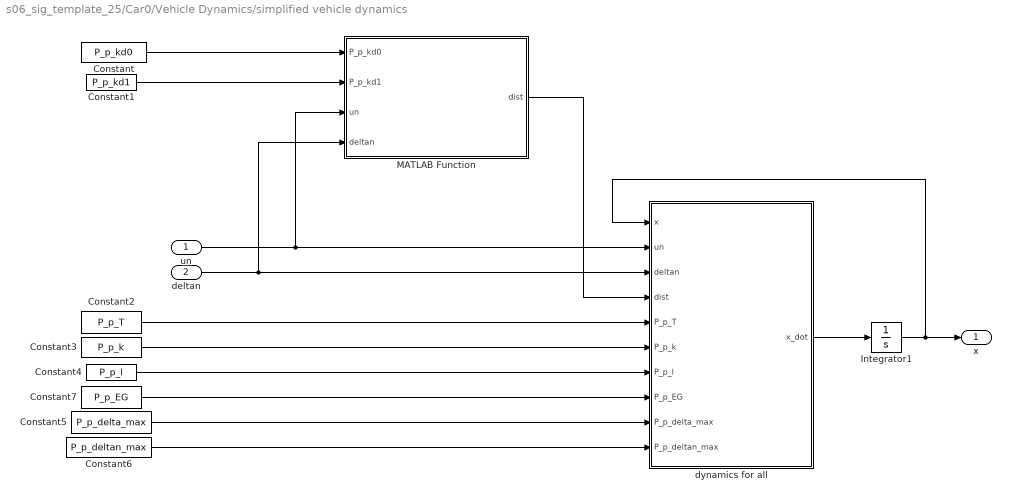
== system s06_sig_template_25/Car0/Vehicle Dynamics/simplified vehicle dynamics ==
  un : Inport
  deltan : Inport  Port=2
  Constant : Constant  Value=P_p_kd0
  Constant1 : Constant  Value=P_p_kd1
  Constant2 : Constant  Value=P_p_T
  Constant3 : Constant  Value=P_p_k
  Constant4 : Constant  Value=P_p_l
  Constant5 : Constant  Value=P_p_delta_max
  Constant6 : Constant  Value=P_p_deltan_max
  Constant7 : Constant  Value=P_p_EG
  Integrator1 : Integrator  InitialCondition=[0;0.5;0.38;0]
  MATLAB Function : MATLAB Function  TreatAsAtomicUnit=on
  dynamics for all : MATLAB Function  TreatAsAtomicUnit=on
  x : Outport
  wires:
  un/1 -> MATLAB Function/3(un), dynamics for all/2(un)
  deltan/1 -> MATLAB Function/4(deltan), dynamics for all/3(deltan)
  MATLAB Function/1(dist) -> dynamics for all/4(dist)
  dynamics for all/1(x_dot) -> Integrator1/1
  Integrator1/1 -> dynamics for all/1(x), x/1
  Constant/1 -> MATLAB Function/1(P_p_kd0)
  Constant1/1 -> MATLAB Function/2(P_p_kd1)
  Constant7/1 -> dynamics for all/8(P_p_EG)
  Constant2/1 -> dynamics for all/5(P_p_T)
  Constant3/1 -> dynamics for all/6(P_p_k)
  Constant4/1 -> dynamics for all/7(P_p_l)
  Constant6/1 -> dynamics for all/10(P_p_deltan_max)
  Constant5/1 -> dynamics for all/9(P_p_delta_max)

== system s06_sig_template_25/Car0/Vehicle Dynamics/vehicle dynamics (continuous, nonlinear) ==
  un : Inport
  deltan : Inport  Port=2
  Integrator1 : Integrator  InitialCondition=[0.5; 0.38; 0; 0; 0; 0; 0]
  MATLAB Function : MATLAB Function  TreatAsAtomicUnit=on
  dynamics for all : MATLAB Function  TreatAsAtomicUnit=on
  x : Outport
  beta : Outport  Port=2
  wires:
  un/1 -> MATLAB Function/1(un), dynamics for all/2(un)  "un"
  deltan/1 -> MATLAB Function/2(deltan), dynamics for all/3(deltan)  "deltan"
  MATLAB Function/1(dist) -> dynamics for all/4(dist)  "dist"
  dynamics for all/1(state_dot) -> Integrator1/1
  Integrator1/1 -> dynamics for all/1(state), x/1
  dynamics for all/2(beta) -> beta/1

== system s06_sig_template_25/Car1/Motion Control/Sliders or Joystick ==
  note: 1) Add Subsystem or Model blocks as valid variant choices.
      | 2) You cannot connect blocks at this level. At simulation, connectivity is automatically
      | determined, based on the active variant and port name matching.
  Joystick : Subsystem  VariantControl=false
  Sliders : Subsystem  VariantControl=true
  action : Outport

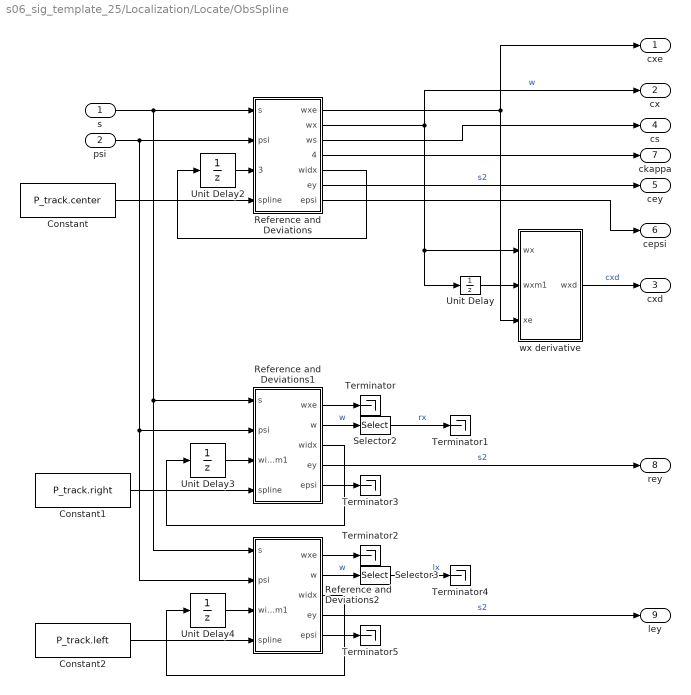
== system s06_sig_template_25/Localization/Locate/ObsSpline ==
  s : Inport
  psi : Inport  Port=2
  Constant : Constant  Value=P_track.center  OutDataTypeStr=Bus: SPLINE
  Constant1 : Constant  Value=P_track.right  OutDataTypeStr=Bus: SPLINE
  Constant2 : Constant  Value=P_track.left  OutDataTypeStr=Bus: SPLINE
  Reference and Deviations : MATLAB Function  TreatAsAtomicUnit=on
  Reference and Deviations1 : MATLAB Function  TreatAsAtomicUnit=on
  Reference and Deviations2 : MATLAB Function  TreatAsAtomicUnit=on
  Selector2 : Selector  InputPortWidth=5  IndexOptions=Index vector (dialog)  Indices=1  OutputSizes=1
  Selector3 : Selector  InputPortWidth=5  IndexOptions=Index vector (dialog)  Indices=1  OutputSizes=1
  Terminator{,1..5} (6 alike) : Terminator
  Unit Delay : UnitDelay  InitialCondition=-1  SampleTime=-1
  Unit Delay2 : UnitDelay  InitialCondition=int32(0)  SampleTime=-1
  Unit Delay3 : UnitDelay  InitialCondition=int32(0)  SampleTime=-1
  Unit Delay4 : UnitDelay  InitialCondition=int32(0)  SampleTime=-1
  wx derivative : MATLAB Function  TreatAsAtomicUnit=on
  cxe : Outport
  cx : Outport  Port=2
  cxd : Outport  Port=3
  cs : Outport  Port=4
  cey : Outport  Port=5
  cepsi : Outport  Port=6
  ckappa : Outport  Port=7
  rey : Outport  Port=8
  ley : Outport  Port=9
  wires:
  Reference and Deviations/6(ey) -> cey/1  "s2"
  Unit Delay/1 -> wx derivative/2(wxm1)
  s/1 -> Reference and Deviations2/1(s), Reference and Deviations1/1(s), Reference and Deviations/1(s)
  Unit Delay2/1 -> Reference and Deviations/3(widxkm1)
  Reference and Deviations/5(widx) -> Unit Delay2/1
  psi/1 -> Reference and Deviations2/2(psi), Reference and Deviations1/2(psi), Reference and Deviations/2(psi)
  Constant/1 -> Reference and Deviations/4(spline)
  Reference and Deviations/7(epsi) -> cepsi/1
  Reference and Deviations/2(wx) -> wx derivative/1(wx), Unit Delay/1, cx/1  "w"
  Reference and Deviations/1(wxe) -> wx derivative/3(xe), cxe/1
  wx derivative/1(wxd) -> cxd/1  "cxd"
  Reference and Deviations/4(wkappa) -> ckappa/1
  Unit Delay3/1 -> Reference and Deviations1/3(widxkm1)
  Reference and Deviations1/3(widx) -> Unit Delay3/1
  Reference and Deviations1/1(wxe) -> Terminator/1
  Reference and Deviations1/2(w) -> Selector2/1  "w"
  Reference and Deviations1/4(ey) -> rey/1  "s2"
  Reference and Deviations1/5(epsi) -> Terminator3/1
  Constant1/1 -> Reference and Deviations1/4(spline)
  Unit Delay4/1 -> Reference and Deviations2/3(widxkm1)
  Constant2/1 -> Reference and Deviations2/4(spline)
  Reference and Deviations2/1(wxe) -> Terminator2/1
  Reference and Deviations2/4(ey) -> ley/1  "s2"
  Reference and Deviations2/3(widx) -> Unit Delay4/1
  Reference and Deviations2/5(epsi) -> Terminator5/1
  Reference and Deviations2/2(w) -> Selector3/1  "w"
  Selector2/1 -> Terminator1/1  "rx"
  Selector3/1 -> Terminator4/1  "lx"
  Reference and Deviations/3(ws) -> cs/1

== system s06_sig_template_25/Car0/Motion Control/Sliders or Joystick/Joystick ==
  Data Type Conversion : DataTypeConversion  OutDataTypeStr=single  SaturateOnIntegerOverflow=off  RndMeth=Floor
  Gain3 : Gain  Gain=-1
  Joystick Input : vrlib/Joystick Input  joyid=1  adjustports=off  forcefeed=off
  Selector1 : Selector  IndexOptions=Index vector (dialog)  Indices=[2 4]  OutputSizes=1
  Terminator : Terminator
  action : Outport
  wires:
  Data Type Conversion/1 -> Selector1/1
  Gain3/1 -> action/1
  Joystick Input/1 -> Data Type Conversion/1
  Selector1/1 -> Gain3/1
  Joystick Input/2 -> Terminator/1

== system s06_sig_template_25/Car0/Motion Control/Sliders or Joystick/Sliders ==
  Gain : Gain  Gain=-1
  Mux1 : Mux  Inputs=2
  Slider : SliderBlock  ScaleMin=-1  ScaleMax=1
  Slider1 : SliderBlock  ScaleMin=-1  ScaleMax=1
  pedals : Constant  Value=single(0.498452)  SampleTime=Inf
  steering : Constant  Value=single(0)
  action : Outport
  wires:
  pedals/1 -> Mux1/1
  Gain/1 -> Mux1/2
  Mux1/1 -> action/1
  steering/1 -> Gain/1

== system s06_sig_template_25/Car1/Motion Control/Sliders or Joystick/Joystick ==
  Data Type Conversion : DataTypeConversion  OutDataTypeStr=single  SaturateOnIntegerOverflow=off  RndMeth=Floor
  Gain3 : Gain  Gain=-1
  Joystick Input : vrlib/Joystick Input  joyid=1  adjustports=off  forcefeed=off
  Selector1 : Selector  IndexOptions=Index vector (dialog)  Indices=[2 4]  OutputSizes=1
  Terminator : Terminator
  action : Outport
  wires:
  Data Type Conversion/1 -> Selector1/1
  Gain3/1 -> action/1
  Joystick Input/1 -> Data Type Conversion/1
  Selector1/1 -> Gain3/1
  Joystick Input/2 -> Terminator/1

== system s06_sig_template_25/Car1/Motion Control/Sliders or Joystick/Sliders ==
  Gain : Gain  Gain=-1
  Mux1 : Mux  Inputs=2
  Slider : SliderBlock  ScaleMin=-1  ScaleMax=1
  Slider1 : SliderBlock  ScaleMin=-1  ScaleMax=1
  pedals : Constant  Value=single(0.4117647)  SampleTime=Inf
  steering : Constant  Value=single(1)
  action : Outport
  wires:
  pedals/1 -> Mux1/1
  Gain/1 -> Mux1/2
  Mux1/1 -> action/1
  steering/1 -> Gain/1

== matlab function s06_sig_template_25/Car0/Motion Control/Refernce Pathfollowing ==
  data: spline input; kappa_star output; v_star output; s_star output; psi_star output; s input; v_ref input; P_p_Tt parameter
function [kappa_star, v_star, s_star,psi_star]   = Reference_pf(spline,s,v_ref,P_p_Tt)
    %decompose bus
    breakslen=spline.breakslen;
    points=spline.points;
    coefs=spline.coefs;
    periodic=spline.periodic;
    
    %get reference (closest points on trajectory)
    [w,~]=mbc_spline_get_reference(s,breakslen,points,coefs,periodic,...
        v_ref,0);
    psi_star=w(2);
    s_star=[w(3);w(4)];
    kappa_star=w(5);
    v_star=v_ref; %v* is needed for lookahead due to deadtime

== matlab function s06_sig_template_25/Car0/Motion Control/Sigma_ref_position ==
  data: v0 input; wp output; xD input; vE input; Y input; Yp input; tE output
function [wp, tE]  = ReferenceSignalGenerator(v0, xD, vE, Y, Yp)

%% Longitudinal position control:
% input
% - v0: velocity at t0; wp'(t0)
% - xD: reference position; wp(tE)-wp(t0); given by maneuver
% - vE: maximum velocity; wp'(tE); given by maneuver
% - Y: current velocity; v(t) for t=[t0;tE]; from carobs % NOTSURE: why do
% i need this?
% - Yp: current (longitudinal) position; yp(t) = x(t); integration of vr from 0 to t
% output
% - Wp: wp(t) as a quintic polynomial; reference for the p controller
% - UVp: feedforward signal

% final goal: target speed of inner control loop Up = URp + UVp = v_star(t)
% reference: slide 7.1 page 5

%% implementation of Longitudinal position control

x0 = 0; % NOTSURE: should we set it here or x0 should be an input?
tE = 5*xD/(3*v0+3*vE);

% wp(t) = c5*t^5 + c4*t^4 + c3*t^3 + c2*t^2 + c1*t + c0
c5 = ( 6*xD  -  3*(v0+vE)*tE  )/(tE^5);
c4 = (-15*xD + (8*v0+7*vE)*tE )/(tE^4);
c3 = ( 10*xD - (6*v0+4*vE)*tE )/(tE^3);
c2 = 0;
c1 = v0;
c0 = x0; % NOTSURE: how and when do we get this x0?
wp = [c0, c1, c2, c3, c4, c5];

== matlab function s06_sig_template_25/Car0/Vehicle Dynamics/additional calculation for outputsext ==
  data: P_p_l input; beta output; deltan input
function beta = fnc_beta(P_p_l, deltan)
% beta: side slip angle

a = P_p_l/2;
beta = atan(a/P_p_l * tan(deltan)); 

end

== matlab function s06_sig_template_25/Car0/Vehicle Dynamics/simplified vehicle dynamics/MATLAB Function ==
  data: P_p_kd0 input; P_p_kd1 input; un input; dist output; deltan input
function dist = disturbance(P_p_kd0,P_p_kd1, un, deltan)

    d_0 = P_p_kd0 + P_p_kd1 * abs(un*deltan);
    
    if un > d_0
        dist = d_0;
    elseif un < -d_0
        dist = -d_0;
    else
        dist = un;
    end

end

== matlab function s06_sig_template_25/Localization/Locate/MATLAB Function ==
  data: matrix input; row output; idx input int32
function row = fcn(matrix, idx)
row = matrix(idx,:);
end

== matlab function s06_sig_template_25/Localization/Locate/outputs ==
  data: v input; z input; yext output size=5
function yext = outputs(v, z) 
%#codegen

psi = z(3);
vabs = sqrt(v(1)*v(1) + v(2)*v(2));
beta = mod(atan2(v(2), v(1)) - psi, 2*pi);
if beta > pi
    beta = beta - 2*pi;
end
if abs(beta) > 0.5 * pi
    vabs = -vabs;
end

yext = [ ...
    z(1) ; ...
    z(2) ; ...
    psi ; ...
    beta ; ...
    vabs ...
    ];
end

== matlab function s06_sig_template_25/Car0/Vehicle Dynamics/vehicle dynamics (continuous, nonlinear)/MATLAB Function ==
  data: un input; dist output; deltan input; P_p_kd0 parameter; P_p_kd1 parameter
function dist = disturbance(un, deltan, P_p_kd0, P_p_kd1)

    d_0 = P_p_kd0 + P_p_kd1 * abs(un*deltan);
    
    if un > d_0
        dist = d_0;
    elseif un < -d_0
        dist = -d_0;
    else
        dist = un;
    end

end

== matlab function s06_sig_template_25/Car0/Vehicle Dynamics/simplified vehicle dynamics/dynamics for all ==
  data: x input; un input; deltan input; dist input; P_p_T input; P_p_k input; P_p_l input; P_p_EG input; P_p_delta_max input; P_p_deltan_max input; x_dot output
function x_dot = vehicle_dynamics(x, un, deltan, dist, P_p_T,P_p_k,P_p_l,P_p_EG,P_p_delta_max,P_p_deltan_max)
    vr = x(1);
    psi = x(4);
    % T = d71_data.P_p_T;
    % k = d71_data.P_p_k;
    % coder.extrinsic('P_p_T');
    % coder.extrinsic('P_p_k');
    dvr = -vr/P_p_T + P_p_k/P_p_T*(un-dist);
    dsr1 = vr * cos(psi);
    dsr2 = vr * sin(psi);
    dpsi = vr/(P_p_l + P_p_EG * vr^2 * sign(vr)) * tan(P_p_delta_max * deltan/P_p_deltan_max);
    x_dot = [dvr; dsr1; dsr2; dpsi];
end

== matlab function s06_sig_template_25/Car0/Vehicle Dynamics/vehicle dynamics (continuous, nonlinear)/dynamics for all ==
  data: state input; un input; deltan input; dist input; state_dot output; beta output; P_p_delta_max parameter; P_p_lf parameter; P_p_lr parameter; P_p_Df parameter; P_p_Dr parameter; P_p_Cf parameter; P_p_Cr parameter; P_p_Bf parameter; P_p_Br parameter; P_p_Ef parameter; P_p_Er parameter; P_p_m parameter; P_p_k parameter; P_p_T parameter; P_p_J parameter; P_p_l parameter; P_p_EG parameter; P_p_deltan_max parameter
function [state_dot,beta] = vehicle_dynamics(state, un, deltan, dist, P_p_delta_max, P_p_lf, P_p_lr, P_p_Df, P_p_Dr, P_p_Cf, P_p_Cr, P_p_Bf, P_p_Br, P_p_Ef, P_p_Er, P_p_m, P_p_k, P_p_T, P_p_J, P_p_l, P_p_EG, P_p_deltan_max)
    
    vc1 = state(3);
    vc1_min = 300; % what should it be?
    if abs(vc1) < vc1_min % use simplified
        vr = state(3); % without slip angle at rear vr = vc1
        psi = state(5);
        dvr = -vr/P_p_T + P_p_k/P_p_T*(un-dist); % this is vc1, and vc2 is 0
        dsr1 = vr * cos(psi);
        dsr2 = vr * sin(psi);

        % safer dpsi computation
        eps_den = 1e-8;        % denominator protection
        eps_deltan = 1e-3;     % your threshold for treating deltan as zero
        tan_arg_limit = 1e2;   % clamp tan argument magnitude to avoid overflow

        if abs(deltan) < eps_deltan
            dpsi = 0;
        else
            % compute denom and protect against zero/near-zero
            denom = P_p_l + P_p_EG .* (vr.^2) .* sign(vr);
            if ~isfinite(denom) || abs(denom) < eps_den
                denom_safe = sign(denom + 1e-16) * eps_den; % preserve sign, avoid 0
            else
                denom_safe = denom;
            end

            % protect P_p_deltan_max
            if ~isfinite(P_p_deltan_max) || abs(P_p_deltan_max) < eps_den
                P_p_deltan_max_safe = sign(P_p_deltan_max + 1e-16) * eps_den;
            else
                P_p_deltan_max_safe = P_p_deltan_max;
            end

            % compute and clamp tan argument
            tan_arg = (P_p_delta_max .* deltan) ./ P_p_deltan_max_safe;
            tan_arg_clamped = max(min(tan_arg, tan_arg_limit), -tan_arg_limit);

            dpsi = (vr ./ denom_safe) .* tan(tan_arg_clamped);
        end


        % dpsi = vr/(P_p_l + P_p_EG * vr^2 * sign(vr)+1e-6) * tan(P_p_delta_max * deltan/P_p_deltan_max);
        omega_dot = 0; % what should it be
        dx = vr;
        state_dot = [dsr1; dsr2; dvr; 0; dpsi; omega_dot; dx];

        % beta function
        a = P_p_l/2;
        beta = atan(a/P_p_l * tan(deltan)); 

    else
        % use the detailed model
        vc1=state(3);
        vc2=state(4);
        psi=state(5);
        psi_dot=state(6);

        delta = P_p_delta_max * deltan;

        if abs(vc1) < 1e-4
            vc1_safe = 1e-4;
        else
            vc1_safe = vc1;
        end
        alpha_f = (-atan((vc2 + P_p_lf * psi_dot)/vc1_safe) + delta) * sign(vc1_safe); % and avoid negative alpha when vc1 is slightly negative
        alpha_r = (-atan((vc2 - P_p_lr * psi_dot)/vc1_safe)) * sign(vc1_safe);

        F_f = P_p_Df * sin(P_p_Cf * atan(P_p_Bf*(1-P_p_Ef)*alpha_f - P_p_Ef * atan(P_p_Bf*alpha_f)));
        F_r = P_p_Dr * sin(P_p_Cr * atan(P_p_Br*(1-P_p_Er)*alpha_r - P_p_Er * atan(P_p_Br*alpha_r)));

        beta = atan2(vc2, vc1);
        s1_dot = vc1 * cos(psi) - vc2 * sin(psi);
        s2_dot = vc1 * sin(psi) + vc2 * cos(psi);
        vc1_dot = 1/P_p_m * (-F_f * sin(delta)+ P_p_m * vc2 * psi_dot)...
            - 1/P_p_T * vc1 + P_p_k*(un - dist) / P_p_T;
        vc2_dot = 1/P_p_m * (F_f * cos(delta) + F_r - P_p_m*vc1*psi_dot);
        omega_dot = 1/P_p_J * (F_f * P_p_lf * cos(delta) - F_r*P_p_lr);
        x_dot = vc1;

        state_dot = [s1_dot; s2_dot; vc1_dot; vc2_dot; psi_dot; omega_dot; x_dot];
    end
end

== matlab function s06_sig_template_25/Car0/Motion Control/Feedforward Pathfollowing ==
  data: kappa_star input; delta_star output; P_p_l parameter
function delta_star = ff_pf(kappa_star, P_p_l)
    delta_star=atan(P_p_l*kappa_star);
